simulink model "cuantizacionSonido"  (R2015a)
settings: Solver=ode45  StartTime=0.0  StopTime=(N-1)/Fs  MaxStep=1/Fs  MinStep=1/Fs  RelTol=1e-3  AbsTol=1/Fs
settings Model: Creator=Javi  LastModifiedBy=Javi
settings SolverCC: InitialStep=1/Fs

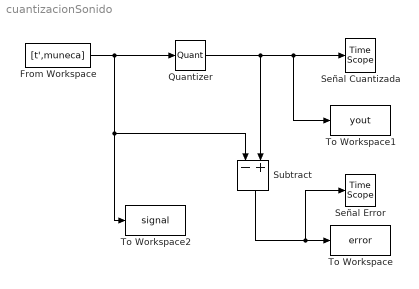
== system cuantizacionSonido ==
  From Workspace : FromWorkspace  VariableName=[t',muneca]  SampleTime=0
  Quantizer : Quantizer  QuantizationInterval=256  LinearizeAsGain=off
  Señal Cuantizada : TimeScope
  Señal Error : TimeScope
  Subtract : Sum  Inputs=-+
  To Workspace : ToWorkspace  VariableName=error  SampleTime=-1
      settings: Save2DSignal=2-D array (concatenate along first dimension)
  To Workspace1 : ToWorkspace  VariableName=yout  SampleTime=-1
      settings: Save2DSignal=2-D array (concatenate along first dimension)
  To Workspace2 : ToWorkspace  VariableName=signal  SampleTime=-1
      settings: Save2DSignal=2-D array (concatenate along first dimension)
  wires:
  Quantizer/1 -> Subtract/2, To Workspace1/1, Señal Cuantizada/1
  From Workspace/1 -> Subtract/1, To Workspace2/1, Quantizer/1
  Subtract/1 -> Señal Error/1, To Workspace/1
